simulink model "System"  (R2022b)
settings: Solver=FixedStepAuto  StartTime=0.0  StopTime=10.0  FixedStep=1e-5  RelTol=1e-3
libraries: arduinolib x2
settings Model: ExtModeTrigDuration=2  Creator=MAAM  LastModifiedBy=MAAM
settings SolverCC: AutoInsertRateTranBlk=on
settings OptimizationCC: DefaultParameterBehavior=Inlined  UseDivisionForNetSlopeComputation=on  GainParamInheritBuiltInType=on  UseFloatMulNetSlope=on  InlineInvariantSignals=on  PassReuseOutputArgsAs=Individual arguments  ZeroExternalMemoryAtStartup=off  ZeroInternalMemoryAtStartup=off  NoFixptDivByZeroProtection=on  EfficientFloat2IntCast=on  LifeSpan=1  MaxStackSize=64  OptimizeBlockOrder=speed  DifferentSizesBufferReuse=on  EfficientTunableParamExpr=on
settings DebuggingCC: ParameterTunabilityLossMsg=error
settings HardwareCC: ProdBitPerInt=16  ProdBitPerPointer=16  ProdBitPerSizeT=16  ProdBitPerPtrDiffT=16  ProdLargestAtomicFloat=None  ProdWordSize=8  ProdLongLongMode=on  ProdHWDeviceType=Atmel->AVR
settings SFSimCC: MATLABDynamicMemAlloc=off
settings RTWCC: Description=Embedded Coder  SystemTargetFile=ert.tlc  HardwareBoard=Arduino Mega 2560  TLCOptions=-aInlineSetEventsForThisBaseRateFcn=TLC_FALSE -aSuppressMultiTaskScheduler=TLC_FALSE -aRateBasedStepFcn=1  TemplateMakefile=ert_default_tmf  Toolchain=Arduino AVR  BuildConfiguration=Faster Runs
settings CodeAppCC: ForceParamTrailComments=on  IgnoreCustomStorageClasses=off  OperatorAnnotations=on  SimulinkDataObjDesc=on  SFDataObjDesc=on  CustomSymbolStrGlobalVar=rt$N$M  CustomSymbolStrType=$N$M  CustomSymbolStrFcn=$N$M$F  CustomSymbolStrMacro=$N$M  InsertBlockDesc=on
settings ERTTargetCC: IncludeMdlTerminateFcn=off  CombineSignalStateStructs=on  SupportComplex=off  SupportContinuousTime=on  ExtModeTransport=3  ExtModeStaticAlloc=on  ExtModeAutomaticAllocSize=off  ExtModeStaticAllocSize=2048  ExtModeMexFile=ext_xcp  ExtModeIntrfLevel=Level2 - Open  InlinedParameterPlacement=NonHierarchical  ERTFilePackagingFormat=CompactWithDataFile

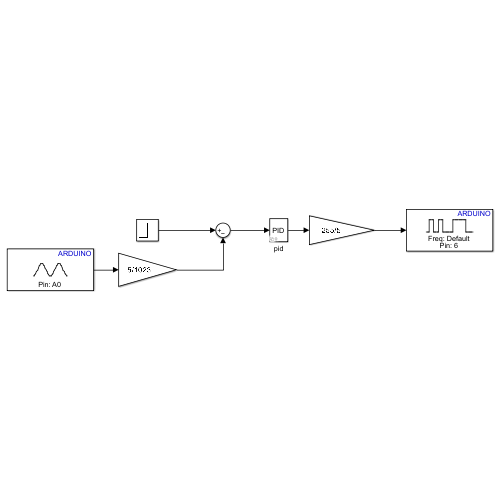
[thumbnail: Simulink's stored preview of the top-level diagram]
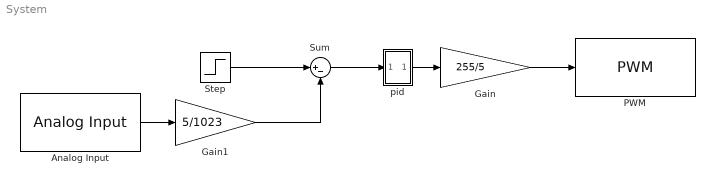
== system System ==
  Analog Input : arduinolib/Analog Input  pinNumber=0  ReadResultsOnly=off  ConversionTriggerSource=Software  ExternalTriggerType=uint32( 0 )  OutputDataType=uint16  EnableConversionCompleteNotify=off  EnableOuputStatus=off  SampleTime=0.0001  blockPlatform=arduino
  Gain : Gain  Gain=255/5  OutDataTypeStr=double
  Gain1 : Gain  Gain=5/1023  OutDataTypeStr=double
  PWM : arduinolib/PWM  pinNumber=6  frequencyType=Default  desiredFrequency=490.2  achievableFrequency=490.2
  Step : Step  SampleTime=0
  Sum : Sum  Inputs=|+-  OutDataTypeStr=double
  pid : Subsystem  Variant=on  mask{F=Parallel, P=10, I=0.1, D=10}
      mask prompts: F "Form"; P "Propotional (P):"; I "Integral      (I):"; D "Drivative    (D):"
      mask init:
      | % Ensure parameters are initialized correctly
      | if isempty(P)
      |     P = 0;
      | end
      | if isempty(I)
      |     I = 0;
      | end
      | if isempty(D)
      |     D = 0;
      | end
      mask TypeOptions F: Parallel | Series | Ideal
      mask TypeOptions P: Subsystem/Gain/Gain | Subsystem1/Gain/Gain | Subsystem2/Gain/Gain
      mask TypeOptions I: Subsystem/Gain1/Gain | Subsystem1/Gain1/Gain | Subsystem2/Gain1/Gain
      mask TypeOptions D: Subsystem/Gain2/Gain | Subsystem1/Gain2/Gain | Subsystem2/Gain2/Gain
      mask Display: fprintf('PID');
  wires:
  pid/1(Out1) -> Gain/1
  Gain/1 -> PWM/1
  Sum/1 -> pid/1(In1)
  Step/1 -> Sum/1
  Analog Input/1 -> Gain1/1
  Gain1/1 -> Sum/2

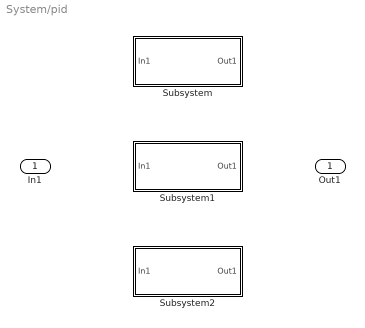
== system System/pid ==
  In1 : Inport
  Subsystem : Subsystem  VariantControl=F==1
  Subsystem1 : Subsystem  VariantControl=F==2
  Subsystem2 : Subsystem  VariantControl=F==3
  Out1 : Outport

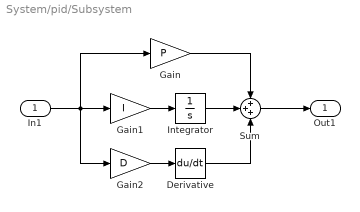
== system System/pid/Subsystem ==
  In1 : Inport
  Derivative : Derivative
  Gain : Gain  Gain=P
  Gain1 : Gain  Gain=I
  Gain2 : Gain  Gain=D
  Integrator : Integrator
  Sum : Sum  Inputs=+++
  Out1 : Outport
  wires:
  Gain1/1 -> Integrator/1
  Gain2/1 -> Derivative/1
  Sum/1 -> Out1/1
  Integrator/1 -> Sum/2
  Gain/1 -> Sum/1
  Derivative/1 -> Sum/3
  In1/1 -> Gain/1, Gain2/1, Gain1/1

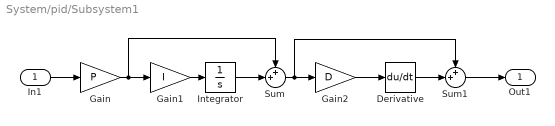
== system System/pid/Subsystem1 ==
  In1 : Inport
  Derivative : Derivative
  Gain : Gain  Gain=P
  Gain1 : Gain  Gain=I
  Gain2 : Gain  Gain=D
  Integrator : Integrator
  Sum : Sum  Inputs=++|
  Sum1 : Sum  Inputs=++|
  Out1 : Outport
  wires:
  Sum/1 -> Sum1/1, Gain2/1
  Gain2/1 -> Derivative/1
  Gain/1 -> Sum/1, Gain1/1
  Integrator/1 -> Sum/2
  Gain1/1 -> Integrator/1
  In1/1 -> Gain/1
  Sum1/1 -> Out1/1
  Derivative/1 -> Sum1/2

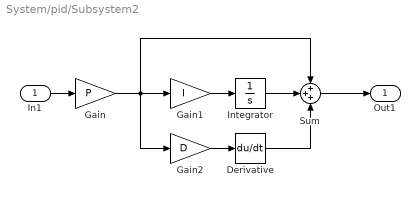
== system System/pid/Subsystem2 ==
  In1 : Inport
  Derivative : Derivative
  Gain : Gain  Gain=P
  Gain1 : Gain  Gain=I
  Gain2 : Gain  Gain=D
  Integrator : Integrator
  Sum : Sum  Inputs=+++
  Out1 : Outport
  wires:
  Gain/1 -> Gain2/1, Gain1/1, Sum/1
  Gain1/1 -> Integrator/1
  Integrator/1 -> Sum/2
  Gain2/1 -> Derivative/1
  Derivative/1 -> Sum/3
  Sum/1 -> Out1/1
  In1/1 -> Gain/1
